simulink model "X8"  (R2015a)
settings: Solver=ode45  StartTime=0.0  StopTime=1000  RelTol=1e-3
values from neighbouring files (symbols this model uses):
  h_ref = 100    [init.m]    (also in initX8_demo.m)
  input_source = 3    [initX8_demo.m]    (also in runX8.m)
  input_source0 = 1    [initX8_demo.m]    (also in runX8.m)
  input_step_time = 0    [initX8_demo.m]    (also in runX8.m = 2)
  lat0 = 37.6205    [init.m]    (also in initX8_demo.m)
  lon0 = -122.3815    [init.m]    (also in initX8_demo.m)
  P = computeGains(T_phi_delta_a,T_v_delta_r,T_theta_delta_e,T_Va_theta,T_Va_delta_t,P)    [initX8_demo.m]
  U_trim = [0.0079    0.0000         0    0.1240]'    [initX8_demo.m]    (also in runX8.m = [0.0079    0.0000         0    0.1240])
  X_trim = [0.0000    0.0000 -150.0000    0.9997    0.0000    0.0232   -0.0000 18.0168    0.0001    0.8366    0.0000    0.0000    0.0000 0.0039 -0.0000    0.0039   -0.0000    0.1240]'    [initX8_demo.m]    (also in runX8.m = x0)
undefined symbols (not defined in the file or in its folder): Earth, F, Kd_phi, Kd_theta, Ki_course, Ki_h, Ki_phi, Ki_V, Kp_course, Kp_h, Kp_phi, Kp_theta, Kp_V, Light, MIL, WGS84, wind, Y_trim
libraries: simulink x9, simulink_extras x6, aerolibfltsims x4, aerolibtransform2 x2, aerolibanimutils x2, aerolibwind2 x2, X8_lib x1
settings Model: CovSFcnEnable=off  Creator=krisgry  LastModifiedBy=krisgry
settings DebuggingCC: SolverPrmCheckMsg=warning  ModelReferenceExtraNoncontSigs=none

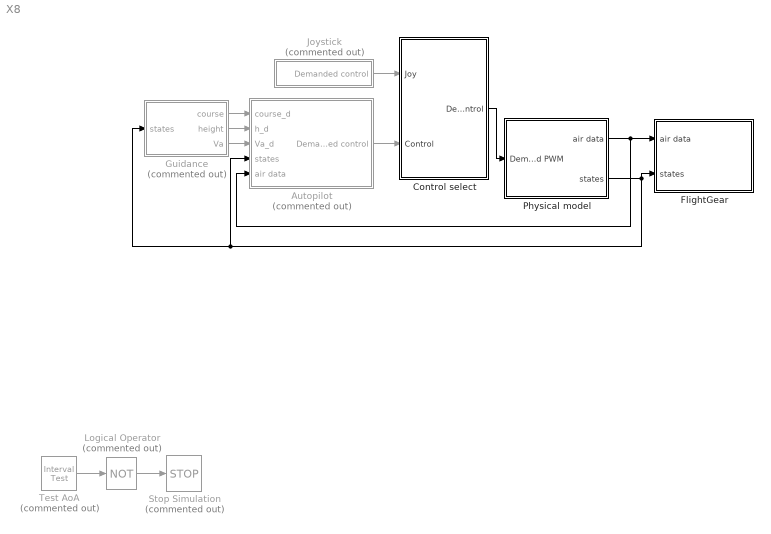
== system X8 ==
  Autopilot : Subsystem  Commented=on
  Control select : Subsystem
  FlightGear : Subsystem
  Guidance : Subsystem  Commented=on
  Joystick : Subsystem  Commented=on
  Logical Operator : Logic  Commented=on  Operator=NOT  AllPortsSameDT=off  OutDataTypeStr=boolean
  Physical model : Subsystem
  Stop Simulation : Stop  Commented=on
  Test AoA : simulink/Logic and Bit Operations/Interval Test  Commented=on  IntervalClosedRight=on  uplimit=15  IntervalClosedLeft=on  lowlimit=-15  OutDataTypeStr=boolean
  wires:
  Physical model/1(air data) -> Autopilot/5(air data), FlightGear/1(air data)
  Test AoA/1 -> Logical Operator/1
  Logical Operator/1 -> Stop Simulation/1
  Physical model/2(states) -> FlightGear/2(states), Guidance/1(states), Autopilot/4(states)
  Guidance/1(course) -> Autopilot/1(course_d)
  Guidance/2(height) -> Autopilot/2(h_d)
  Guidance/3(Va) -> Autopilot/3(Va_d)
  Joystick/1(Demanded control) -> Control select/1(Joy)
  Autopilot/1(Demanded control) -> Control select/2(Control)
  Control select/1(Demanded control) -> Physical model/1(Demanded PWM)

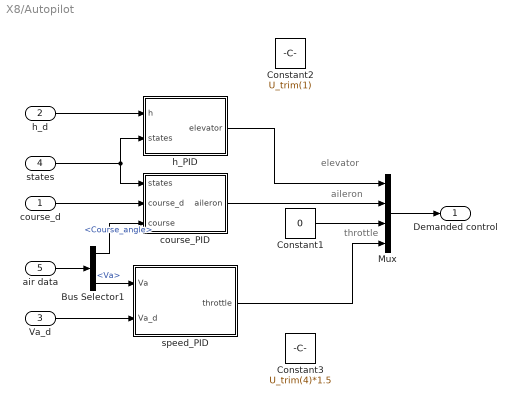
== system X8/Autopilot ==
  note: throttle
  note: aileron
  note: elevator
  course_d : Inport
  h_d : Inport  Port=2
  Va_d : Inport  Port=3
  states : Inport  Port=4
  air data : Inport  Port=5
  Bus Selector1 : BusSelector  OutputSignals=Course_angle,Path_angle,Va
  Constant1 : Constant  Value=0
  Constant2 : Constant  Value=U_trim(1)
  Constant3 : Constant  Value=U_trim(4)*1.5
  Mux : Mux
  course_PID : Subsystem
  h_PID : Subsystem
  speed_PID : Subsystem
  Demanded control : Outport
  wires:
  Mux/1 -> Demanded control/1
  states/1 -> h_PID/2(states), course_PID/1(states)
  Constant1/1 -> Mux/3
  air data/1 -> Bus Selector1/1
  h_d/1 -> h_PID/1(h)
  course_d/1 -> course_PID/2(course_d)
  Bus Selector1/1 -> course_PID/3(course)  "<Course_angle>"
  course_PID/1(aileron) -> Mux/2
  Bus Selector1/3 -> speed_PID/1(Va)  "<Va>"
  Va_d/1 -> speed_PID/2(Va_d)
  speed_PID/1(throttle) -> Mux/4
  h_PID/1(elevator) -> Mux/1

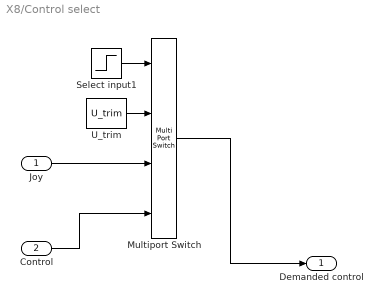
== system X8/Control select ==
  Joy : Inport
  Control : Inport  Port=2
  Multiport Switch : MultiPortSwitch
  Select input1 : Step  Time=input_step_time  Before=input_source0  After=input_source  SampleTime=0
  U_trim : Constant  Value=U_trim
  Demanded control : Outport
  wires:
  Control/1 -> Multiport Switch/4
  Multiport Switch/1 -> Demanded control/1
  U_trim/1 -> Multiport Switch/2
  Joy/1 -> Multiport Switch/3
  Select input1/1 -> Multiport Switch/1

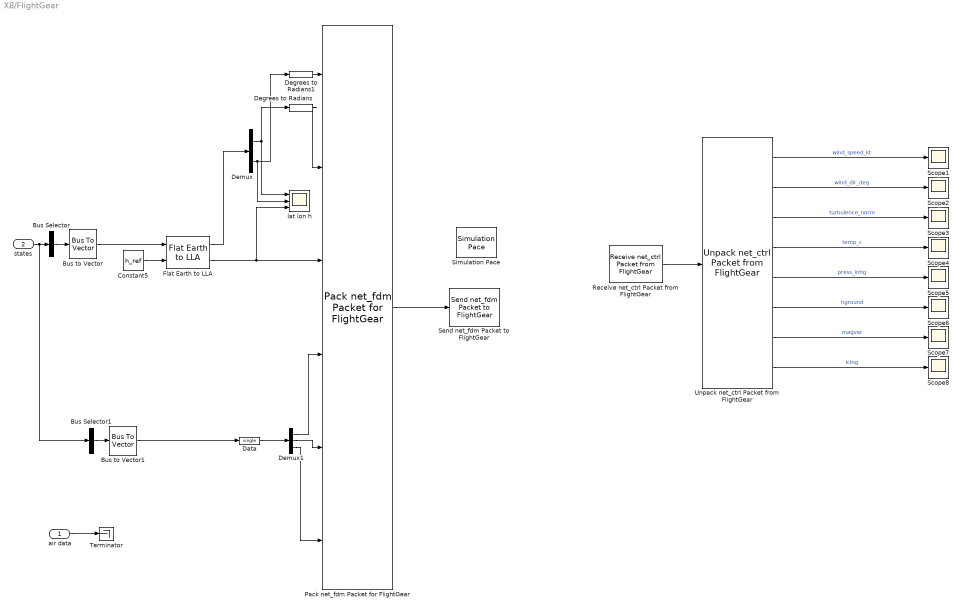
== system X8/FlightGear ==
  air data : Inport
  states : Inport  Port=2
  Bus Selector : BusSelector  OutputSignals=Position.p_N,Position.p_E,Position.p_D  OutputAsBus=on
  Bus Selector1 : BusSelector  OutputSignals=Attitude  OutputAsBus=on
  Bus to Vector : BusToVector
  Bus to Vector1 : BusToVector
  Constant5 : Constant  Value=h_ref
  Data : DataTypeConversion  OutDataTypeStr=single
  Degrees to Radians : simulink_extras/Transformations/Degrees to Radians
  Degrees to Radians1 : simulink_extras/Transformations/Degrees to Radians
  Demux : Demux  Outputs=2
  Demux1 : Demux  Outputs=3
  Flat Earth to LLA : aerolibtransform2/Flat Earth to LLA  units=Metric (MKS)  ptype=Earth (WGS84)  F=1/298.257223563  R=6378137  LL0=[lat0 lon0]  psi=0
  Pack net_fdm Packet for FlightGear : aerolibfltsims/Pack net_fdm Packet for FlightGear  FlightGearVersion=v2.12  ShowPositionAttitudeInputs=on  ShowVelocityAccelerationInputs=off  ShowControlSurfacePositionInputs=off  ShowEngineFuelInputs=off  ShowLandingGearInputs=off  ShowEnvironmentInputs=off  SampleTime=1/30
  Receive net_ctrl Packet from FlightGear : aerolibfltsims/Receive net_ctrl Packet from FlightGear  FlightGearVersion=v2.12  ReceiveAddress=129.241.154.119  ReceivePort=5505  ReceiveWidth=744  varLen=off  SampleTime=1/30  packetFlag=off
      settings: AttributesFormatString=Version Selected:\n%<FlightGearVersion>
  Scope{1..8} (8 alike) : Scope
      Scope1 settings: YMin=3  YMax=3  SaveName=ScopeData16
      Scope3 settings: SaveName=ScopeData2
      Scope4 settings: YMin=14.1217  YMax=14.1217  SaveName=ScopeData3
      Scope5 settings: YMin=29.9199  YMax=29.9199  SaveName=ScopeData4
      Scope6 settings: SaveName=ScopeData5
      Scope7 settings: SaveName=ScopeData6
      Scope8 settings: SaveName=ScopeData7
  Send net_fdm Packet to FlightGear : aerolibfltsims/Send net_fdm Packet to FlightGear  DestinationIpAddress=129.241.154.119  DestinationPort=5502  LocalIpPort=-1  varLen=off  SampleTime=1/30
  Simulation Pace : aerolibanimutils/Simulation Pace  SimulationPace=1  SleepMode=MATLAB Thread  OutputPaceError=off  SampleTime=1/30
      settings: AttributesFormatString=%<SimulationPace> sec/sec
  Terminator : Terminator
  Unpack net_ctrl Packet from FlightGear : aerolibfltsims/Unpack net_ctrl Packet from FlightGear  FlightGearVersion=v2.12  ShowControlSurfacePositionOutputs=off  ShowEngineFuelOutputs=off  ShowLandingGearOutputs=off  ShowAvionicOutputs=off  ShowEnvironmentOutputs=on  SampleTime=1/30
      settings: AttributesFormatString=Version Selected: %<FlightGearVersion>
  lat lon h : Scope  NumInputPorts=3
      settings: YMin=37.6205~-122.382~-3  YMax=37.6238~-122.381~1  SaveName=ScopeData17
  wires:
  Pack net_fdm Packet for FlightGear/1 -> Send net_fdm Packet to FlightGear/1
  Demux1/1 -> Pack net_fdm Packet for FlightGear/4
  Demux1/2 -> Pack net_fdm Packet for FlightGear/5
  Demux1/3 -> Pack net_fdm Packet for FlightGear/6
  Demux/2 -> lat lon h/2, Degrees to Radians1/1
  Demux/1 -> Degrees to Radians/1, lat lon h/1
  Data/1 -> Demux1/1
  Degrees to Radians/1 -> Pack net_fdm Packet for FlightGear/2
  Degrees to Radians1/1 -> Pack net_fdm Packet for FlightGear/1
  Unpack net_ctrl Packet from FlightGear/1 -> Scope1/1  "wind_speed_kt"
  Receive net_ctrl Packet from FlightGear/1 -> Unpack net_ctrl Packet from FlightGear/1
  Unpack net_ctrl Packet from FlightGear/2 -> Scope2/1  "wind_dir_deg"
  Unpack net_ctrl Packet from FlightGear/3 -> Scope3/1  "turbulence_norm"
  Unpack net_ctrl Packet from FlightGear/4 -> Scope4/1  "temp_c"
  Unpack net_ctrl Packet from FlightGear/5 -> Scope5/1  "press_inhg"
  Unpack net_ctrl Packet from FlightGear/6 -> Scope6/1  "hground"
  Unpack net_ctrl Packet from FlightGear/7 -> Scope7/1  "magvar"
  Unpack net_ctrl Packet from FlightGear/8 -> Scope8/1  "icing"
  air data/1 -> Terminator/1
  Constant5/1 -> Flat Earth to LLA/2
  Flat Earth to LLA/1 -> Demux/1
  Bus Selector/1 -> Bus to Vector/1
  Bus to Vector/1 -> Flat Earth to LLA/1
  Flat Earth to LLA/2 -> lat lon h/3, Pack net_fdm Packet for FlightGear/3
  Bus Selector1/1 -> Bus to Vector1/1
  Bus to Vector1/1 -> Data/1
  states/1 -> Bus Selector1/1, Bus Selector/1

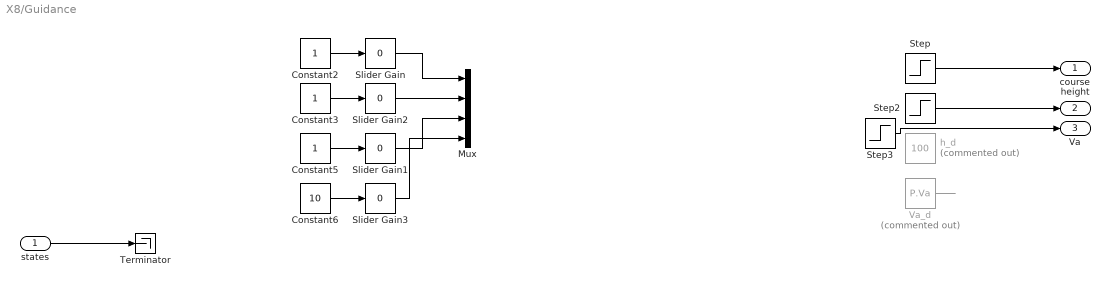
== system X8/Guidance ==
  states : Inport
  Constant2 : Constant
  Constant3 : Constant
  Constant5 : Constant
  Constant6 : Constant  Value=10
  Mux : Mux
  Slider Gain : simulink/Math Operations/Slider Gain  low=-10  gain=0  high=10
  Slider Gain1 : simulink/Math Operations/Slider Gain  low=-1  gain=0  high=1
  Slider Gain2 : simulink/Math Operations/Slider Gain  low=0  gain=0  high=1
  Slider Gain3 : simulink/Math Operations/Slider Gain  low=-1  gain=0  high=1
  Step : Step  Time=0  Before=X_trim(4)  After=X_trim(4)  SampleTime=0
  Step2 : Step  Time=10  Before=100  After=100  SampleTime=0
  Step3 : Step  Before=Y_trim(1)  After=Y_trim(1)+4  SampleTime=0
  Terminator : Terminator
  Va_d : Constant  Commented=on  Value=P.Va
  h_d : Constant  Commented=on  Value=100
  course : Outport
  height : Outport  Port=2
  Va : Outport  Port=3
  wires:
  Va_d/1 -> ?
  Step/1 -> course/1
  Step2/1 -> height/1
  Step3/1 -> Va/1
  Constant2/1 -> Slider Gain/1
  Constant3/1 -> Slider Gain2/1
  Constant5/1 -> Slider Gain1/1
  Constant6/1 -> Slider Gain3/1
  Slider Gain/1 -> Mux/1
  Slider Gain2/1 -> Mux/2
  Slider Gain1/1 -> Mux/3
  Slider Gain3/1 -> Mux/4
  states/1 -> Terminator/1

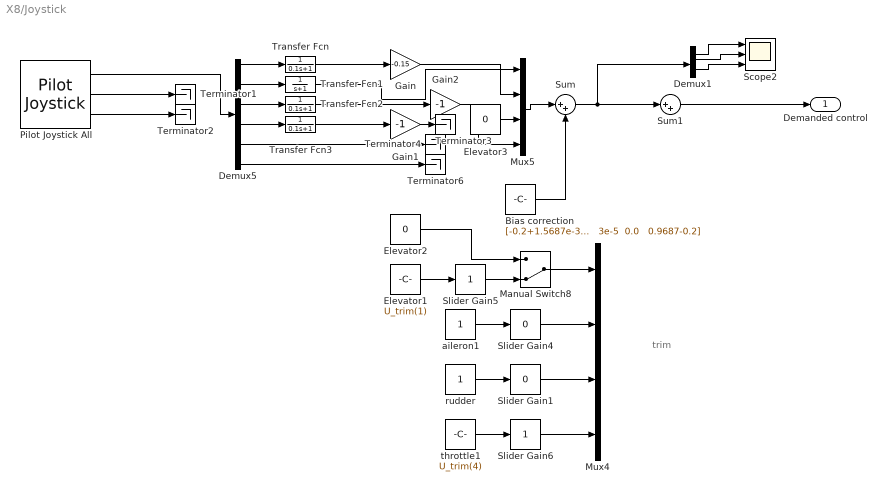
== system X8/Joystick ==
  note: trim
  Bias correction : Constant  Value="[-0.2+1.5687e-3   3e-5  0.0   0.9687-0.2]"
  Demux1 : Demux
  Demux5 : Demux  Outputs=6
  Elevator1 : Constant  Value=U_trim(1)
  Elevator2 : Constant  Value=0
  Elevator3 : Constant  Value=0
  Gain : Gain  Gain=-0.15
  Gain1 : Gain  Gain=-1
  Gain2 : Gain  Gain=-1
  Manual Switch8 : ManualSwitch  CurrentSetting=0
  Mux4 : Mux
  Mux5 : Mux
  Pilot Joystick All : aerolibanimutils/Pilot Joystick  JoystickID=Joystick1  OutputConfiguration=AllOutputs  SampleTime=1/30
  Scope2 : Scope  NumInputPorts=3
      settings: YMin=-0.16~2.54e-05~-0.025  YMax=-2.77556e-17~2.575e-05~0.35  SaveName=ScopeData18
  Slider Gain1 : simulink/Math Operations/Slider Gain  low=-1  gain=0  high=1
  Slider Gain4 : simulink/Math Operations/Slider Gain  low=-1  gain=0  high=1
  Slider Gain5 : simulink/Math Operations/Slider Gain  low=-1  gain=1  high=1
  Slider Gain6 : simulink/Math Operations/Slider Gain  low=0  gain=1  high=2
  Sum : Sum  Inputs=|++
  Sum1 : Sum  Inputs=|++
  Terminator{1..4,6} (5 alike) : Terminator
  Transfer Fcn : TransferFcn  Denominator=[0.1 1]
  Transfer Fcn1 : TransferFcn  Denominator=[1 1]
  Transfer Fcn2 : TransferFcn  Denominator=[0.1 1]
  Transfer Fcn3 : TransferFcn  Denominator=[0.1 1]
  aileron1 : Constant
  rudder : Constant
  throttle1 : Constant  Value=U_trim(4)
  Demanded control : Outport
  wires:
  Gain/1 -> Mux5/2
  Demux5/5 -> Terminator4/1
  Demux5/1 -> Transfer Fcn/1
  Demux5/6 -> Terminator6/1
  Demux5/4 -> Transfer Fcn3/1
  Pilot Joystick All/3 -> Terminator2/1
  Pilot Joystick All/2 -> Terminator1/1
  Gain1/1 -> Terminator3/1
  Demux5/3 -> Transfer Fcn2/1
  Mux5/1 -> Sum/1
  Bias correction/1 -> Sum/2
  Gain2/1 -> Mux5/4
  Demux1/1 -> Scope2/1
  Demux1/2 -> Scope2/2
  Sum/1 -> Sum1/1, Demux1/1
  Elevator1/1 -> Slider Gain5/1
  aileron1/1 -> Slider Gain4/1
  Slider Gain4/1 -> Mux4/2
  Slider Gain6/1 -> Mux4/4
  Manual Switch8/1 -> Mux4/1
  Slider Gain5/1 -> Manual Switch8/2
  Elevator2/1 -> Manual Switch8/1
  Sum1/1 -> Demanded control/1
  throttle1/1 -> Slider Gain6/1
  Demux1/4 -> Scope2/3
  Elevator3/1 -> Mux5/3
  rudder/1 -> Slider Gain1/1
  Slider Gain1/1 -> Mux4/3
  Demux5/2 -> Transfer Fcn1/1
  Pilot Joystick All/1 -> Demux5/1
  Transfer Fcn/1 -> Gain/1
  Transfer Fcn1/1 -> Mux5/1
  Transfer Fcn2/1 -> Gain2/1
  Transfer Fcn3/1 -> Gain1/1

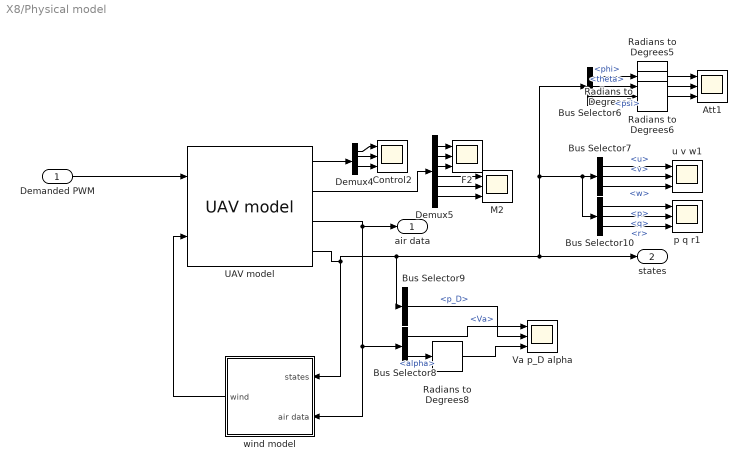
== system X8/Physical model ==
  Demanded PWM : Inport
  Att1 : Scope  NumInputPorts=3
      settings: ShowLegends=on  TimeRange=18  YMin=-15~-20~-80  YMax=55~45~120  SaveName=ScopeData27
  Bus Selector10 : BusSelector  OutputSignals=AngularVelocity.p,AngularVelocity.q,AngularVelocity.r
  Bus Selector6 : BusSelector  OutputSignals=Attitude.phi,Attitude.theta,Attitude.psi
  Bus Selector7 : BusSelector  OutputSignals=Velocity.u,Velocity.v,Velocity.w
  Bus Selector8 : BusSelector  OutputSignals=Va,alpha
  Bus Selector9 : BusSelector  OutputSignals=Position.p_D
  Control2 : Scope  NumInputPorts=3
      settings: YMin=0.00799684~2.03634e-07~0.100994  YMax=0.00883862~2.2507e-07~0.111624  SaveName=ScopeData28
  Demux4 : Demux
  Demux5 : Demux  Outputs=6
  F2 : Scope  NumInputPorts=3
      settings: YMin=-30~-3~-150  YMax=55~5~70  SaveName=ScopeData29
  M2 : Scope  NumInputPorts=3
      settings: YMin=0.0078~-0.0185~-0.0175  YMax=0.0091~-0.0125~-0.01425  SaveName=ScopeData30
  Radians to Degrees{5..8} (4 alike) : simulink_extras/Transformations/Radians to Degrees
  UAV model : X8_lib/UAV model  param='x8_param'  pos0=[0,0,0]  quat0=[1,0,0,0]  vel0=[0,0,0]  rate0=[0,0,0]  servoR_pos0=0  servoR_vel0=0  servoL_pos0=0  servoL_vel0=0  prop_speed0=0
  Va p_D alpha : Scope  NumInputPorts=3
      settings: TimeRange=1000  YMin=12.75~-130~3.65  YMax=17.5~-125.5~4.75  SaveName=ScopeData31
  p q r1 : Scope  NumInputPorts=3
      settings: YMin=-1~-1.5~-4  YMax=2.25~2.75~1.5  SaveName=ScopeData32
  u v w1 : Scope  NumInputPorts=3
      settings: YMin=12.25~-6e-05~1.03  YMax=17.75~2e-05~1.13  SaveName=ScopeData33
  wind model : Subsystem
  air data : Outport
  states : Outport  Port=2
  wires:
  Demux5/1 -> F2/1
  Demux5/2 -> F2/2
  Demux5/3 -> F2/3
  Demux5/4 -> M2/1
  Demux5/5 -> M2/2
  Demux5/6 -> M2/3
  Bus Selector7/1 -> u v w1/1  "<u>"
  Bus Selector7/2 -> u v w1/2  "<v>"
  Bus Selector7/3 -> u v w1/3  "<w>"
  Bus Selector6/1 -> Radians to Degrees5/1  "<phi>"
  Bus Selector6/3 -> Radians to Degrees7/1  "<psi>"
  Bus Selector6/2 -> Radians to Degrees6/1  "<theta>"
  Radians to Degrees5/1 -> Att1/1
  Radians to Degrees6/1 -> Att1/2
  Radians to Degrees7/1 -> Att1/3
  Bus Selector8/1 -> Va p_D alpha/1  "<Va>"
  Bus Selector9/1 -> Va p_D alpha/2  "<p_D>"
  Bus Selector8/2 -> Radians to Degrees8/1  "<alpha>"
  Radians to Degrees8/1 -> Va p_D alpha/3
  Demux4/4 -> Control2/3
  Demux4/2 -> Control2/2
  Demux4/1 -> Control2/1
  Bus Selector10/1 -> p q r1/1  "<p>"
  Bus Selector10/2 -> p q r1/2  "<q>"
  Bus Selector10/3 -> p q r1/3  "<r>"
  UAV model/3 -> air data/1, Bus Selector8/1, wind model/2(air data)
  UAV model/4 -> Bus Selector9/1, Bus Selector6/1, Bus Selector7/1, Bus Selector10/1, states/1, wind model/1(states)
  UAV model/2 -> Demux5/1
  Demanded PWM/1 -> UAV model/1
  wind model/1(wind) -> UAV model/2
  UAV model/1 -> Demux4/1

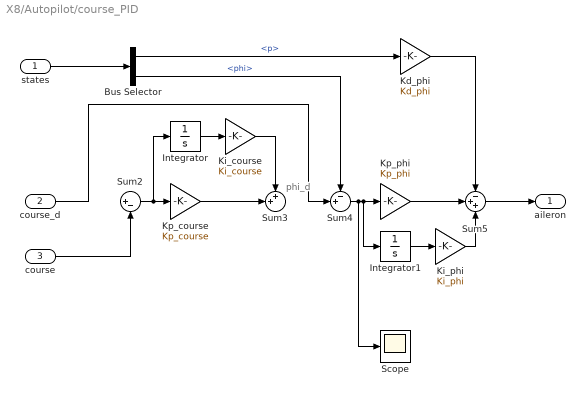
== system X8/Autopilot/course_PID ==
  note: phi_d
  states : Inport
  course_d : Inport  Port=2
  course : Inport  Port=3
  Bus Selector : BusSelector  OutputSignals=AngularVelocity.p,Attitude.phi
  Integrator : Integrator
  Integrator1 : Integrator  LimitOutput=on  UpperSaturationLimit=0.7  LowerSaturationLimit=-0.7
  Kd_phi : Gain  Gain=Kd_phi
  Ki_course : Gain  Gain=Ki_course
  Ki_phi : Gain  Gain=Ki_phi
  Kp_course : Gain  Gain=Kp_course
  Kp_phi : Gain  Gain=Kp_phi
  Scope : Scope
      settings: YMin=0.5  YMax=8  SaveName=ScopeData11
  Sum2 : Sum  Inputs=|+-
  Sum3 : Sum  Inputs=++|
  Sum4 : Sum  Inputs=-+|
  Sum5 : Sum  Inputs=-++
  aileron : Outport
  wires:
  Sum2/1 -> Integrator/1, Kp_course/1
  Bus Selector/1 -> Kd_phi/1  "<p>"
  Bus Selector/2 -> Sum4/1  "<phi>"
  Sum5/1 -> aileron/1
  course/1 -> Sum2/2
  Integrator/1 -> Ki_course/1
  Kp_course/1 -> Sum3/2
  Kd_phi/1 -> Sum5/1
  Ki_course/1 -> Sum3/1
  Sum4/1 -> Scope/1, Integrator1/1, Kp_phi/1
  Integrator1/1 -> Ki_phi/1
  Kp_phi/1 -> Sum5/2
  Ki_phi/1 -> Sum5/3
  states/1 -> Bus Selector/1
  course_d/1 -> Sum4/2

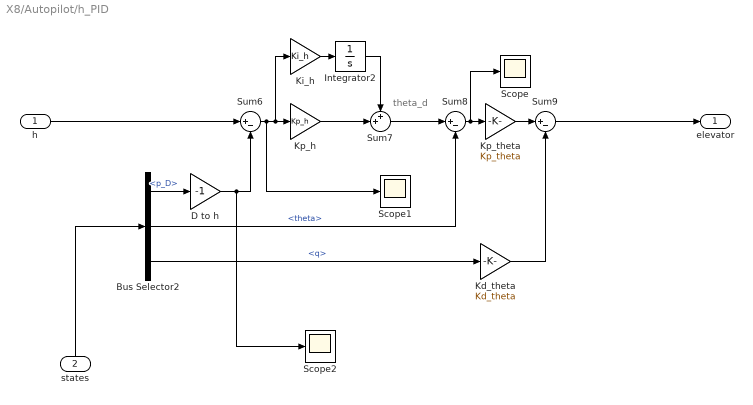
== system X8/Autopilot/h_PID ==
  note: theta_d
  h : Inport
  states : Inport  Port=2
  Bus Selector2 : BusSelector  OutputSignals=Position.p_D,Attitude.theta,AngularVelocity.q
  D to h : Gain  Gain=-1
  Integrator2 : Integrator  LimitOutput=on  UpperSaturationLimit=1  LowerSaturationLimit=-1
  Kd_theta : Gain  Gain=Kd_theta
  Ki_h : Gain  Gain=Ki_h
  Kp_h : Gain  Gain=Kp_h
  Kp_theta : Gain  Gain=Kp_theta
  Scope : Scope
      settings: YMin=0.004  YMax=0.01  SaveName=ScopeData12
  Scope1 : Scope
      settings: YMin=0.75  YMax=2.75  SaveName=ScopeData13
  Scope2 : Scope
      settings: YMin=98  YMax=101  SaveName=ScopeData14
  Sum6 : Sum  Inputs=|+-
  Sum7 : Sum  Inputs=++|
  Sum8 : Sum  Inputs=|+-
  Sum9 : Sum  Inputs=|+-
  elevator : Outport
  wires:
  Sum9/1 -> elevator/1
  Sum6/1 -> Scope1/1, Ki_h/1, Kp_h/1
  Sum8/1 -> Scope/1, Kp_theta/1
  Bus Selector2/3 -> Kd_theta/1  "<q>"
  Integrator2/1 -> Sum7/1
  D to h/1 -> Scope2/1, Sum6/2
  Kp_h/1 -> Sum7/2
  Bus Selector2/1 -> D to h/1  "<p_D>"
  states/1 -> Bus Selector2/1
  Kp_theta/1 -> Sum9/1
  Kd_theta/1 -> Sum9/2
  Bus Selector2/2 -> Sum8/2  "<theta>"
  h/1 -> Sum6/1
  Ki_h/1 -> Integrator2/1
  Sum7/1 -> Sum8/1

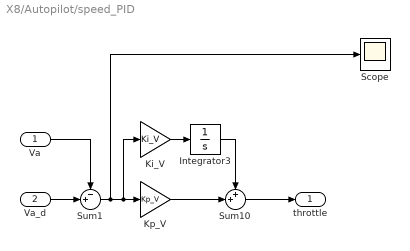
== system X8/Autopilot/speed_PID ==
  Va : Inport
  Va_d : Inport  Port=2
  Integrator3 : Integrator  LimitOutput=on  UpperSaturationLimit=1  LowerSaturationLimit=0
  Ki_V : Gain  Gain=Ki_V
  Kp_V : Gain  Gain=Kp_V
  Scope : Scope
      settings: YMin=-2.5  YMax=20  SaveName=ScopeData15
  Sum1 : Sum  Inputs=-+|
  Sum10 : Sum  Inputs=++|
  throttle : Outport
  wires:
  Va/1 -> Sum1/1
  Sum10/1 -> throttle/1
  Ki_V/1 -> Integrator3/1
  Va_d/1 -> Sum1/2
  Kp_V/1 -> Sum10/2
  Sum1/1 -> Scope/1, Ki_V/1, Kp_V/1
  Integrator3/1 -> Sum10/1

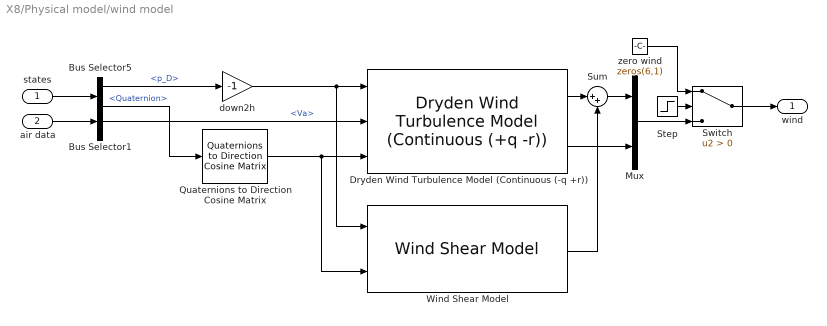
== system X8/Physical model/wind model ==
  states : Inport
  air data : Inport  Port=2
  Bus Selector1 : BusSelector  OutputSignals=Va
  Bus Selector5 : BusSelector  OutputSignals=Position.p_D,Quaternion
  Dryden Wind Turbulence Model (Continuous (-q +r)) : aerolibwind2/Dryden Wind Turbulence Model  (Continuous (+q -r))  units=Metric (MKS)  spec=MIL-F-8785C  model=Continuous Dryden (-q +r)  W20=wind.speed  Wdeg=wind.dir  TurbProb=10^-2 - Light  L_high=533.4  Wingspan=P.b  ts=0.1  Seed=[23341 23342 23343 23344]  T_on=on
  Mux : Mux  Inputs=2
  Quaternions to Direction Cosine Matrix : aerolibtransform2/Quaternions to  Direction Cosine Matrix
  Step : Step  Time=wind.start_time  Before=1  After=0  SampleTime=0
  Sum : Sum  Inputs=|++
  Switch : Switch  Criteria=u2 > Threshold
  Wind Shear Model : aerolibwind2/Wind Shear Model  units=Metric (MKS)  phase=Category C - Terminal Flight Phase  W_20=wind.speed  Wdeg=wind.dir
  down2h : Gain  Gain=-1
  zero wind : Constant  Value=zeros(6,1)
  wind : Outport
  wires:
  Bus Selector5/1 -> down2h/1  "<p_D>"
  Quaternions to Direction Cosine Matrix/1 -> Wind Shear Model/2, Dryden Wind Turbulence Model (Continuous (-q +r))/3
  Bus Selector1/1 -> Dryden Wind Turbulence Model (Continuous (-q +r))/2  "<Va>"
  Dryden Wind Turbulence Model (Continuous (-q +r))/2 -> Mux/2
  zero wind/1 -> Switch/1
  Switch/1 -> wind/1
  Bus Selector5/2 -> Quaternions to Direction Cosine Matrix/1  "<Quaternion>"
  air data/1 -> Bus Selector1/1
  states/1 -> Bus Selector5/1
  down2h/1 -> Wind Shear Model/1, Dryden Wind Turbulence Model (Continuous (-q +r))/1
  Step/1 -> Switch/2
  Mux/1 -> Switch/3
  Dryden Wind Turbulence Model (Continuous (-q +r))/1 -> Sum/1
  Sum/1 -> Mux/1
  Wind Shear Model/1 -> Sum/2
